simulink model "design_project_fuzzy_bmw"  (R2018a)
settings: Solver=VariableStepAuto  StartTime=0.0  StopTime=120  RelTol=1e-3
libraries: simulink x2, fuzblock x1, simulink_extras x1
settings Model: Creator=DELL  LastModifiedBy=DELL

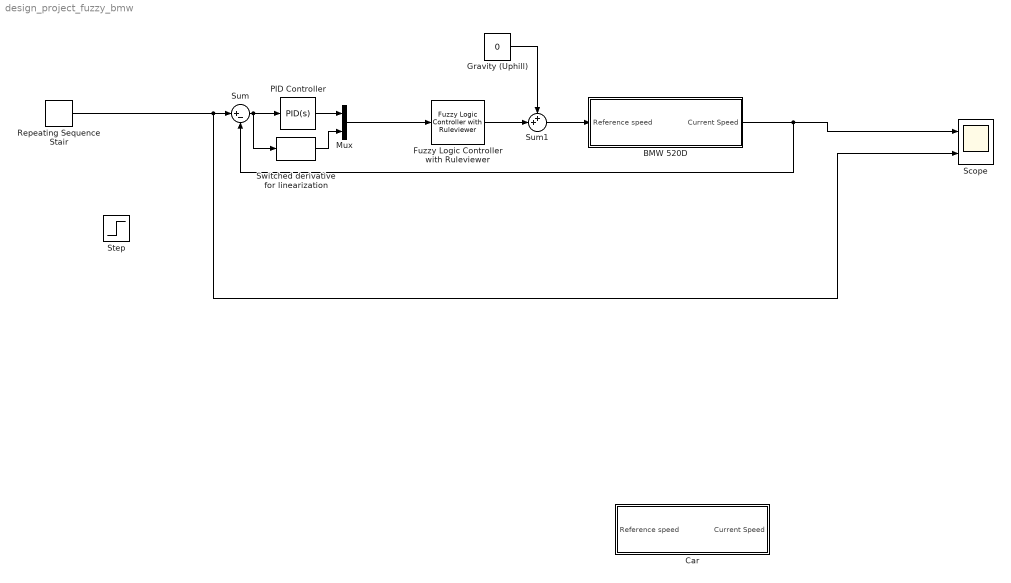
== system design_project_fuzzy_bmw ==
  BMW 520D : Subsystem
  Car : Subsystem
  Fuzzy Logic Controller with Ruleviewer : fuzblock/Fuzzy Logic  Controller  with Ruleviewer  fismatrix=rules_gauss_mf_bmw_520d  Ts=1
  "Gravity (Uphill) " : Constant  Value=0
  Mux : Mux  Inputs=2
  PID Controller : simulink/Continuous/PID Controller  Controller=PID  TimeDomain=Continuous-time  SampleTime=-1  IntegratorMethod=Forward Euler  FilterMethod=Forward Euler  Form=Parallel  UseFilter=on  ControllerParametersSource=internal  P=100  I=0  D=0  N=100  InitialConditionSource=internal  InitialConditionForIntegrator=0  InitialConditionForFilter=0  ExternalReset=none  LimitOutput=on  UpperSaturationLimit=110  LowerSaturationLimit=-110  LinearizeAsGain=on  AntiWindupMode=none  Kb=1  TrackingMode=off  Kt=1  PParamMin=[]  PParamMax=[]  IParamMin=[]  IParamMax=[]  DParamMin=[]  DParamMax=[]  NParamMin=[]  NParamMax=[]  KbParamMin=[]  KbParamMax=[]  KtParamMin=[]  KtParamMax=[]  POutMin=[]  POutMax=[]  IOutMin=[]  IOutMax=[]  DOutMin=[]  DOutMax=[]  NOutMin=[]  NOutMax=[]  KbOutMin=[]  KbOutMax=[]  KtOutMin=[]  KtOutMax=[]  IntegratorOutMin=[]  IntegratorOutMax=[]  FilterOutMin=[]  FilterOutMax=[]  SumOutMin=[]  SumOutMax=[]  SumI1OutMin=[]  SumI1OutMax=[]  SumI2OutMin=[]  SumI2OutMax=[]  SumI3OutMin=[]  SumI3OutMax=[]  SumDOutMin=[]  SumDOutMax=[]  SaturationOutMin=[]  SaturationOutMax=[]  IntegratorContinuousStateAttributes=''  IntegratorStateMustResolveToSignalObject=off  IntegratorRTWStateStorageClass=Auto  FilterContinuousStateAttributes=''  FilterStateMustResolveToSignalObject=off  FilterRTWStateStorageClass=Auto  DifferentiatorICPrevScaledInput=0  DifferentiatorOutMin=[]  DifferentiatorOutMax=[]  FilterDiffOutCoefMin=[]  FilterDiffOutCoefMax=[]  SumDenOutMin=[]  SumDenOutMax=[]  SumNumOutMin=[]  SumNumOutMax=[]  ReciprocalOutMin=[]  ReciprocalOutMax=[]  DivideOutMin=[]  DivideOutMax=[]  TunerSelectOption=Transfer Function Based (PID Tuner App)
  Repeating Sequence Stair : simulink/Sources/Repeating Sequence Stair  OutValues=[10 20 40 80 110 90 60 30 10]  tsamp=8  OutMin=[]  OutMax=[]  OutDataTypeStr=int8  OutputDataTypeScalingMode=int8  OutDataType=fixdt(0,8)  ConRadixGroup=Best Precision: Vector-wise  OutScaling=2^-12
  Scope : Scope  NumInputPorts=2
  Step : Step  Time=0  After=100  SampleTime=0
  Sum : Sum  Inputs=|+-
  Sum1 : Sum  Inputs=++|
  Switched derivative for linearization : simulink_extras/Linearization/Switched derivative for linearization  switchVal=0  derivConst=100
      settings: SourceProductName=Simulink  SourceProductBaseCode=SL
  wires:
  BMW 520D/1(Current Speed) -> Sum/2, Scope/1
  Fuzzy Logic Controller with Ruleviewer/1 -> Sum1/2
  Mux/1 -> Fuzzy Logic Controller with Ruleviewer/1
  Switched derivative for linearization/1 -> Mux/2
  Repeating Sequence Stair/1 -> Scope/2, Sum/1
  Sum1/1 -> BMW 520D/1(Reference speed)
  "Gravity (Uphill) "/1 -> Sum1/1
  Sum/1 -> PID Controller/1, Switched derivative for linearization/1
  PID Controller/1 -> Mux/1

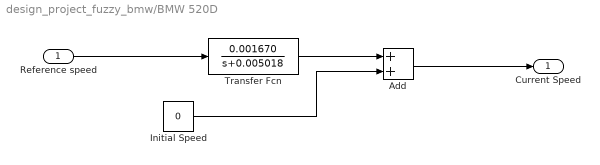
== system design_project_fuzzy_bmw/BMW 520D ==
  Reference speed : Inport
  Add : Sum
  Initial Speed : Constant  Value=0
  Transfer Fcn : TransferFcn  Numerator=[0.001670]  Denominator=[1 0.005018]
  Current Speed : Outport
  wires:
  Initial Speed/1 -> Add/2
  Add/1 -> Current Speed/1
  Reference speed/1 -> Transfer Fcn/1
  Transfer Fcn/1 -> Add/1

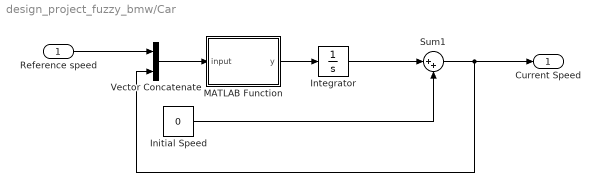
== system design_project_fuzzy_bmw/Car ==
  Reference speed : Inport
  Initial Speed : Constant  Value=0
  Integrator : Integrator
  MATLAB Function : MATLAB Function  TreatAsAtomicUnit=on
  Sum1 : Sum  Inputs=|++
  Vector Concatenate : Concatenate
  Current Speed : Outport
  wires:
  Initial Speed/1 -> Sum1/2
  Reference speed/1 -> Vector Concatenate/1
  Sum1/1 -> Current Speed/1, Vector Concatenate/2
  Vector Concatenate/1 -> MATLAB Function/1(input)
  MATLAB Function/1(y) -> Integrator/1
  Integrator/1 -> Sum1/1

== matlab function design_project_fuzzy_bmw/Car/MATLAB Function ==
  data: input input; y output
function y = cruise_control(input)
y = (0.001 * input(2) - 0.3*1.18*0.72* input(1));
% y = (input (2) - 0.3 * input(1)); 
end
